simulink model "Simulation"  (R2022a)
settings: Solver=VariableStepAuto  StartTime=0.0  StopTime=10  FixedStep=0.001  RelTol=1e-3
model workspace (MAT data in the model file):
  A = 1
values from neighbouring files (symbols this model uses):
  I = 1    [Simulation1.m]
  M = 1    [Simulation1.m]    (also in map.mat = [0 0 0 0 0 0 0 0 0 0 0 0 ... (3145728 elements, 1024x1024x3); provaReds.m = [1   0   0     0      0        0; splitandcolor.m = 255 * repmat(uint8(map.value), 1, 1, 3))
  v0x = vXp(1)    [Simulation1.m]    (also in interTornambe.m = vxp(1); provaReds.m = vxp(1))
  v0y = vYp(1)    [Simulation1.m]    (also in provaReds.m = vyp(1))
  x0 = w1(1)    [Simulation1.m]    (also in interTornambe.m = xp(1); provaReds.m = xp(1))
  y0 = w2(1)    [Simulation1.m]    (also in provaReds.m = yp(1))
undefined symbols (not defined in the file or in its folder): omega0, theta0
libraries: dspsrcs4 x6
settings Model: Creator=loryb  LastModifiedBy=loryb

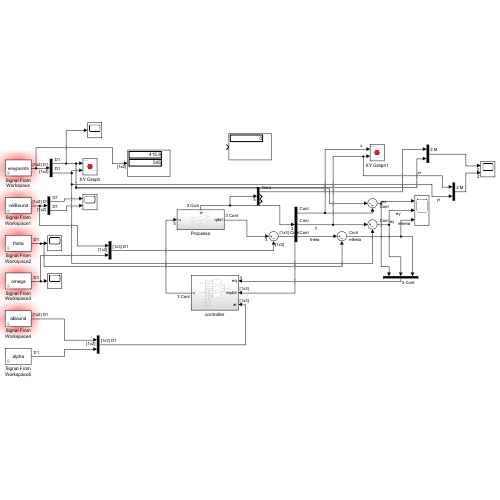
[thumbnail: Simulink's stored preview of the top-level diagram]
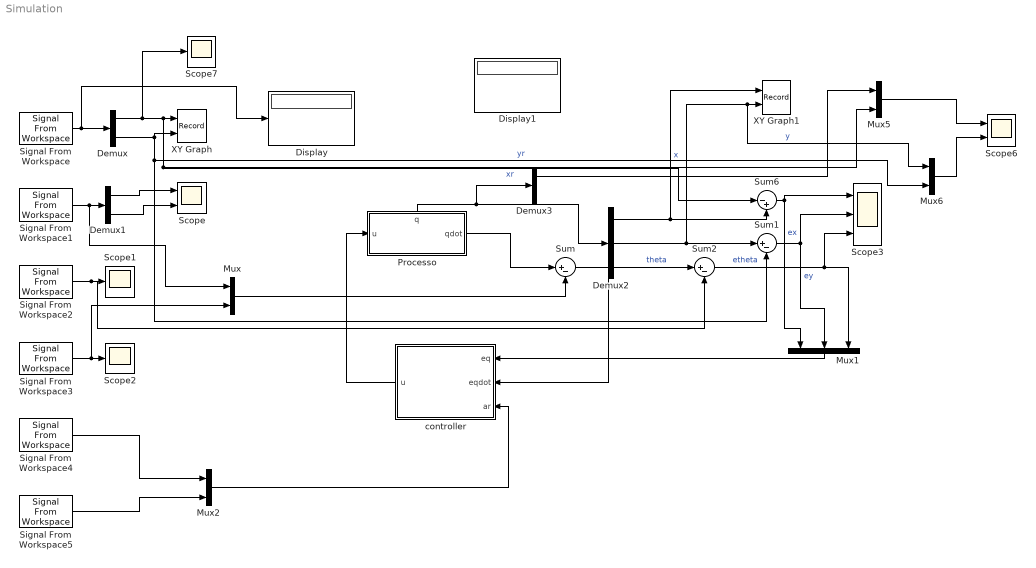
== system Simulation ==
  Demux : Demux  Outputs=2
  Demux1 : Demux  Outputs=2
  Demux2 : Demux  Outputs=3
  Demux3 : Demux  Outputs=3
  Display : Display
  Display1 : Display
  Mux{,2,5..6} (4 alike) : Mux  Inputs=2
  Mux1 : Mux  Inputs=3
  Processo : Subsystem
      settings: PortSchema="{\"entries\":[{\"content\":{\"sides\":[{\"content\":{\"connectorIds\":[\"In1\"]},\"type\":\"ConnectorPlacement.EquallySpacedRectSide\",\"uuid\":\"453c70f7-8eef-41b4-b37e-2425462fd600\"},{\"content\":{\"connectorIds\":[\"Out1\"],\"side\":\"RIGHT\"},\"type\":\"ConnectorPlacement.EquallySpacedRectSide\",\"uuid\":\"7333ccd7-0dc8-412c-b4a2-ce8ef9332ba0\"},{\"content\":{\"connectorIds\":[\"Out2\"],\"side\":\"TOP\"},\"type\":\"ConnectorPlacement.EquallySpacedRectSide\",\"uuid\":\"2a73c39c-f43d-46cc-8895-98ea3e6953d1\"}]},\"type\":\"ConnectorPlacement.EquallySpacedConnector\",\"uuid\":\"5f23e24f-fb88-4846-8a4a-b3c01d22b663\"}],\"packageUris\":[\"http://schema.mathworks.com/mf0/Connector/R2020b\"],\"version\":\"1.0\"}"
  Scope : Scope  NumInputPorts=2
  Scope1 : Scope
  Scope2 : Scope
  Scope3 : Scope  NumInputPorts=3
  Scope6 : Scope  NumInputPorts=2
  Scope7 : Scope
  Signal From Workspace : dspsrcs4/Signal From Workspace  X=waypoints  Ts=1e-3  nsamps=1  OutputAfterFinalValue=Holding final value  ignoreOrWarnInputAndFrameLengths=off  OutputFrames=off
  Signal From Workspace1 : dspsrcs4/Signal From Workspace  X=velBound  Ts=1e-3  nsamps=1  OutputAfterFinalValue=Setting to zero  ignoreOrWarnInputAndFrameLengths=off  OutputFrames=off
  Signal From Workspace2 : dspsrcs4/Signal From Workspace  X=theta  Ts=1e-3  nsamps=1  OutputAfterFinalValue=Holding final value  ignoreOrWarnInputAndFrameLengths=off  OutputFrames=off
  Signal From Workspace3 : dspsrcs4/Signal From Workspace  X=omega  Ts=1e-3  nsamps=1  OutputAfterFinalValue=Setting to zero  ignoreOrWarnInputAndFrameLengths=off  OutputFrames=off
  Signal From Workspace4 : dspsrcs4/Signal From Workspace  X=aBound  Ts=1e-3  nsamps=1  OutputAfterFinalValue=Setting to zero  ignoreOrWarnInputAndFrameLengths=off  OutputFrames=off
  Signal From Workspace5 : dspsrcs4/Signal From Workspace  X=alpha  Ts=1e-3  nsamps=1  OutputAfterFinalValue=Setting to zero  ignoreOrWarnInputAndFrameLengths=off  OutputFrames=off
  Sum : Sum  Inputs=|+-
  Sum1 : Sum  Inputs=|+-
  Sum2 : Sum  Inputs=|+-
  Sum6 : Sum  Inputs=|-+
  XY Graph : Record  FileSettingsInternal="{\"entries\":[{\"content\":{\"excelSettings\":{\"content\":{},\"type\":\"Streamout.ExcelSettings\"}},\"type\":\"Streamout.FileSettingStorage\",\"uuid\":\"83ab58d6-1a90-44e5-b866-a4710f50015f\"}],\"packageUris\":[\"http://schema.mathworks.com/mf0/streamout_blocks/R2020a\"],\"version\":\"1.0\"}"  Layout=[1 1]  SignalsInternal="{\"entries\":[{\"content\":{\"signals\":[{\"content\":{\"blockPath\":[\"Simulation/XY Graph\"],\"channel\":[],\"dimensions\":[1,1],\"domain\":\"Simulation/XY Graph\",\"lineColor\":\"#a2142f\",\"plots\":[1],\"port\":1,\"sid\":[\"\"],\"signalID\":16175,\"signalName\":\"xr\"},\"type\":\"RecordBlkView.Signal\",\"uuid\":\"57dcfea6-0348-44d7-931f-cc0569265494\"},{\"content\":{\"blockPath\":[\"Simulation/XY Graph\"],\"channel\":[],\"dimensions\":[1,1],\"domain\":\"Simulation/XY Graph\",\"lineColor\":\"#139fff\",\"plots\":[1],\"port\":2,\"sid\":[\"\"],\"signalID\":16179,\"signalName\":\"yr\"},\"type\":\"RecordBlkView.Signal\",\"uuid\":\"e21958f7-f0de-4ac0-a4f3-bd680d062655\"}]},\"type\":\"RecordBlkView.InputSignals\",\"uuid\":\"7f752984-92ea-4d1d-83ae-591a31dfe649\"}],\"packageUris\":[\"http://schema.mathworks.com/mf0/streamout_blocks/R2020a\"],\"version\":\"1.0\"}"  VisualizationBindings="{\"xyplotplugin\":{\"info\":[{\"series\":[{\"bindingParametersList\":[{\"parameter\":\"X-Axis\",\"signalID\":16175,\"signalName\":\"xr\"},{\"parameter\":\"Y-Axis\",\"signalID\":16179,\"signalName\":\"yr\"}],\"seriesID\":24407}],\"subplotID\":1}]}}"  CompatibilityTag=XY  st=-1
  XY Graph1 : Record  FileSettingsInternal="{\"entries\":[{\"content\":{\"excelSettings\":{\"content\":{},\"type\":\"Streamout.ExcelSettings\"}},\"type\":\"Streamout.FileSettingStorage\",\"uuid\":\"6bc1ff7e-0137-4bff-ad49-5e41b2e0eda7\"}],\"packageUris\":[\"http://schema.mathworks.com/mf0/streamout_blocks/R2020a\"],\"version\":\"1.0\"}"  Layout=[1 1]  SignalsInternal="{\"entries\":[{\"content\":{\"signals\":[{\"content\":{\"blockPath\":[\"Simulation/XY Graph1\"],\"channel\":[],\"dimensions\":[1],\"domain\":\"Simulation/XY Graph1\",\"lineColor\":\"#a2142f\",\"plots\":[1],\"port\":1,\"sid\":[\"\"],\"signalID\":16183,\"signalName\":\"x\"},\"type\":\"RecordBlkView.Signal\",\"uuid\":\"72753513-3c58-4c7a-aff6-1fda32093746\"},{\"content\":{\"blockPath\":[\"Simulation/XY Graph1\"],\"channel\":[],\"dimensions\":[1],\"domain\":\"Simulation/XY Graph1\",\"lineColor\":\"#139fff\",\"plots\":[1],\"port\":2,\"sid\":[\"\"],\"signalID\":16187,\"signalName\":\"y\"},\"type\":\"RecordBlkView.Signal\",\"uuid\":\"3637747b-dcf7-404f-a0d5-798782377fda\"}]},\"type\":\"RecordBlkView.InputSignals\",\"uuid\":\"50e04b57-a542-4ccd-ae11-803c99ffcaac\"}],\"packageUris\":[\"http://schema.mathworks.com/mf0/streamout_blocks/R2020a\"],\"version\":\"1.0\"}"  VisualizationBindings="{\"xyplotplugin\":{\"info\":[{\"series\":[{\"bindingParametersList\":[{\"parameter\":\"X-Axis\",\"signalID\":16183,\"signalName\":\"x\"},{\"parameter\":\"Y-Axis\",\"signalID\":16187,\"signalName\":\"y\"}],\"seriesID\":49458}],\"subplotID\":1}]}}"  CompatibilityTag=XY  st=-1
  controller : Subsystem
  wires:
  Signal From Workspace/1 -> Display/1, Demux/1
  Demux/1 -> Scope7/1, Sum6/1, Mux5/2, XY Graph/1  "xr"
  Demux/2 -> Sum1/2, Mux6/2, XY Graph/2  "yr"
  Signal From Workspace1/1 -> Mux/1, Demux1/1
  Demux1/1 -> Scope/1
  Demux1/2 -> Scope/2
  Signal From Workspace2/1 -> Sum2/2, Scope1/1
  Signal From Workspace3/1 -> Mux/2, Scope2/1
  Signal From Workspace4/1 -> Mux2/1
  Signal From Workspace5/1 -> Mux2/2
  Mux2/1 -> controller/3(ar)
  Demux2/1 -> XY Graph1/1, Sum6/2  "x"
  Demux2/2 -> Mux6/1, XY Graph1/2, Sum1/1  "y"
  Demux2/3 -> Sum2/1  "theta"
  Sum6/1 -> Scope3/1, Mux1/1  "ex"
  Sum1/1 -> Scope3/2, Mux1/2  "ey"
  Sum2/1 -> Scope3/3, Mux1/3  "etheta"
  Mux1/1 -> controller/1(eq)
  Mux/1 -> Sum/2
  Sum/1 -> controller/2(eqdot)
  Mux5/1 -> Scope6/1
  Mux6/1 -> Scope6/2
  controller/1(u) -> Processo/1(u)
  Processo/2(q) -> Demux3/1, Demux2/1
  Processo/1(qdot) -> Sum/1
  Demux3/1 -> Mux5/1

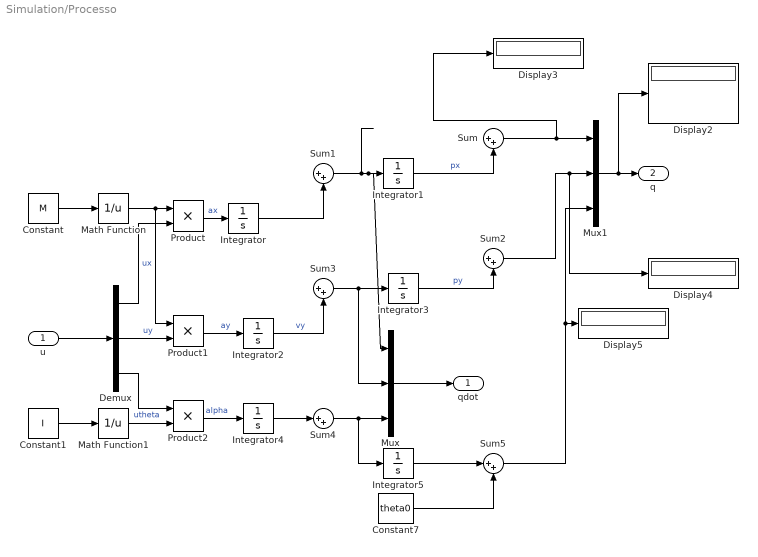
== system Simulation/Processo ==
  u : Inport
  Constant : Constant  Value=M
  Constant1 : Constant  Value=I
  Constant7 : Constant  Value=theta0
  Demux : Demux  Outputs=3
  Display{2..5} (4 alike) : Display
  Integrator : Integrator  InitialCondition=v0x
  Integrator1 : Integrator  InitialCondition=x0
  Integrator2 : Integrator  InitialCondition=v0y
  Integrator3 : Integrator  InitialCondition=y0
  Integrator4 : Integrator  InitialCondition=omega0
  Integrator5 : Integrator  InitialCondition=theta0
  Math Function : Math  Operator=reciprocal
  Math Function1 : Math  Operator=reciprocal
  Mux : Mux  Inputs=3
  Mux1 : Mux  Inputs=3
  Product : Product
  Product1 : Product
  Product2 : Product
  Sum{,1..5} (6 alike) : Sum  Inputs=|++
  qdot : Outport
  q : Outport  Port=2
  wires:
  Sum5/1 -> Display5/1, Mux1/3
  Sum3/1 -> Integrator3/1, Mux/2
  Integrator5/1 -> Sum5/1
  Constant7/1 -> Sum5/2
  Demux/1 -> Product/2  "ux"
  Demux/3 -> Product2/1  "utheta"
  Integrator4/1 -> Sum4/1
  Demux/2 -> Product1/2  "uy"
  Product2/1 -> Integrator4/1  "alpha"
  Sum2/1 -> Display4/1, Mux1/2
  Product1/1 -> Integrator2/1  "ay"
  Sum/1 -> Display3/1, Mux1/1
  Sum1/1 -> Integrator1/1, Mux/1
  Math Function1/1 -> Product2/2
  Constant1/1 -> Math Function1/1
  Integrator1/1 -> Sum/2  "px"
  Integrator2/1 -> Sum3/2  "vy"
  Integrator3/1 -> Sum2/2  "py"
  Mux/1 -> qdot/1
  Product/1 -> Integrator/1  "ax"
  Math Function/1 -> Product1/1, Product/1
  u/1 -> Demux/1
  Constant/1 -> Math Function/1
  Sum4/1 -> Mux/3, Integrator5/1
  Mux1/1 -> Display2/1, q/1
  Integrator/1 -> Sum1/2
  ? -> Sum/1
  ? -> Sum3/1

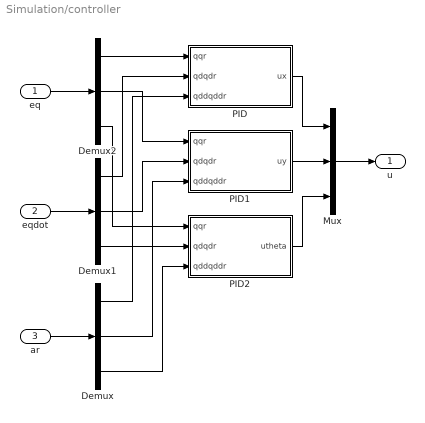
== system Simulation/controller ==
  eq : Inport
  eqdot : Inport  Port=2
  ar : Inport  Port=3
  Demux : Demux  Outputs=3
  Demux1 : Demux  Outputs=3
  Demux2 : Demux  Outputs=3
  Mux : Mux  Inputs=3
  PID : Subsystem
  PID1 : Subsystem
  PID2 : Subsystem
  u : Outport
  wires:
  Demux/3 -> PID2/3(qddqddr)
  Demux/1 -> PID/3(qddqddr)
  Demux/2 -> PID1/3(qddqddr)
  eq/1 -> Demux2/1
  Demux1/1 -> PID/2(qdqdr)
  Demux1/2 -> PID1/2(qdqdr)
  Demux1/3 -> PID2/2(qdqdr)
  Demux2/2 -> PID1/1(qqr)
  Demux2/3 -> PID2/1(qqr)
  Demux2/1 -> PID/1(qqr)
  ar/1 -> Demux/1
  eqdot/1 -> Demux1/1
  PID2/1(utheta) -> Mux/3
  PID1/1(uy) -> Mux/2
  PID/1(ux) -> Mux/1
  Mux/1 -> u/1

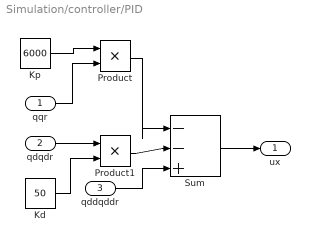
== system Simulation/controller/PID ==
  qqr : Inport
  qdqdr : Inport  Port=2
  qddqddr : Inport  Port=3
  Kd : Constant  Value=50
  Kp : Constant  Value=6000
  Product : Product
  Product1 : Product
  Sum : Sum  Inputs=|--+
  ux : Outport
  wires:
  Sum/1 -> ux/1
  Kp/1 -> Product/1
  qdqdr/1 -> Product1/1
  qddqddr/1 -> Sum/3
  Kd/1 -> Product1/2
  Product/1 -> Sum/1
  Product1/1 -> Sum/2
  qqr/1 -> Product/2

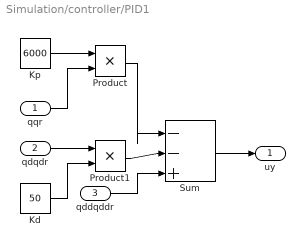
== system Simulation/controller/PID1 ==
  qqr : Inport
  qdqdr : Inport  Port=2
  qddqddr : Inport  Port=3
  Kd : Constant  Value=50
  Kp : Constant  Value=6000
  Product : Product
  Product1 : Product
  Sum : Sum  Inputs=|--+
  uy : Outport
  wires:
  qqr/1 -> Product/2
  Kp/1 -> Product/1
  qdqdr/1 -> Product1/1
  Kd/1 -> Product1/2
  Product/1 -> Sum/1
  qddqddr/1 -> Sum/3
  Product1/1 -> Sum/2
  Sum/1 -> uy/1

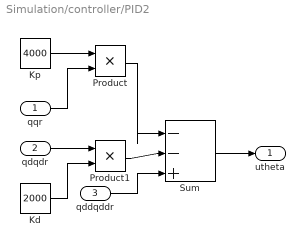
== system Simulation/controller/PID2 ==
  qqr : Inport
  qdqdr : Inport  Port=2
  qddqddr : Inport  Port=3
  Kd : Constant  Value=2000
  Kp : Constant  Value=4000
  Product : Product
  Product1 : Product
  Sum : Sum  Inputs=|--+
  utheta : Outport
  wires:
  Kp/1 -> Product/1
  Product/1 -> Sum/1
  Product1/1 -> Sum/2
  Sum/1 -> utheta/1
  qqr/1 -> Product/2
  qdqdr/1 -> Product1/1
  Kd/1 -> Product1/2
  qddqddr/1 -> Sum/3
